simulink model "sldemo_wheelspeed_absbrake"  (R2020b)
settings: Solver=ode45  StartTime=0.0  StopTime=25  MaxStep=.01  RelTol=1e-3  AbsTol=1e-6
model workspace (MAT data in the model file):
  I = 5
  Kf = 1
  PBmax = 1500
  Rr = 1.25
  TB = 0.01
  v0 = 88
settings Model: ExtModeTrigMode=oneshot  ExtModeArmWhenConnect=off  ExtModeAutoUpdateStatusClock=off  Creator=WELCOME  LastModifiedBy=WELCOME
settings SolverCC: AutoScaleAbsTol=off
settings DataIOCC: SaveFormat=Array  SaveOutput=off  SaveTime=off  ReturnWorkspaceOutputs=off  TimeSaveName=time
settings OptimizationCC: DefaultParameterBehavior=Inlined  InlineInvariantSignals=on  ExpressionDepthLimit=2147483647  InitFltsAndDblsToZero=on  LifeSpan=inf  BufferReusableBoundary=off
settings DebuggingCC: SaveWithParameterizedLinksMsg=none  MultiTaskDSMMsg=warning  SigSpecEnsureSampleTimeMsg=none  IntegerOverflowMsg=none  FcnCallInpInsideContextMsg=warning  BusObjectLabelMismatch=none  ModelReferenceSymbolNameMessage=none  StateNameClashWarn=warning  SFUnexpectedBacktrackingDiag=warning  SFNoUnconditionalDefaultTransitionDiag=warning  SFExecutionAtInitializationDiag=none  IntegerSaturationMsg=none  ArithmeticOperatorsInVariantConditions=warning
settings HardwareCC: ProdBitPerPointer=32  ProdBitPerSizeT=32  ProdBitPerPtrDiffT=32  ProdLargestAtomicFloat=None  ProdIntDivRoundTo=Undefined  ProdEndianess=Unspecified  ProdWordSize=32  ProdHWDeviceType=32-bit Generic  TargetBitPerPointer=64  TargetBitPerSizeT=64  TargetBitPerPtrDiffT=64  TargetLongLongMode=on  TargetIntDivRoundTo=Zero  TargetEndianess=LittleEndian  TargetWordSize=64  TargetHWDeviceType=MATLAB Host
settings ModelReferenceCC: ModelReferenceMinAlgLoopOccurrences=on  PropagateSignalLabelsOutOfModel=off
settings SFSimCC: SimUseLocalCustomCode=off  CustomCodeUndefinedFunction=UseInterfaceOnly
settings RTWCC: Description=Rapid Simulation Target  SystemTargetFile=rsim.tlc  TemplateMakefile=rsim_default_tmf  RTWUseLocalCustomCode=off
settings CodeAppCC: StateflowObjectComments=on
settings RSimTargetCC: TargetFcnLib=ansi_tfl_tmw.mat
settings ConfigComp: CovMetricSettings=dw  CovSaveCumulativeToWorkspaceVar=on  CovSaveSingleToWorkspaceVar=on  CovExternalEMLEnable=off

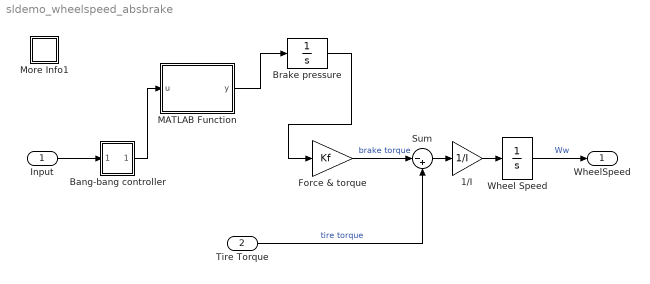
== system sldemo_wheelspeed_absbrake ==
  Input : Inport  SampleTime=0
  Tire Torque : Inport  Port=2
  1/I : Gain  Gain=1/I  SaturateOnIntegerOverflow=on  OutDataTypeStr=Inherit: Same as input  ParamDataTypeStr=Inherit: Same as input
  Bang-bang controller : Subsystem  mask(Sign){}
      mask help: y = sign(x)
      mask Help: Sign Function:\n\t\t\ty = 1 if x > 0\n\t\t\ty = 0 if x = 0\n\t\t\ty = -1 if x < 0
      mask Display: plot(-50,-50,50,50,[-50,50],[0,0],[0,0],[-50,50],[-40,0],[-30,-30],[0,40],[30,30])
  Brake pressure : Integrator  LimitOutput=on  UpperSaturationLimit=PBmax  LowerSaturationLimit=0
  Force & torque : Gain  Gain=Kf  SaturateOnIntegerOverflow=on  OutDataTypeStr=Inherit: Same as input  ParamDataTypeStr=Inherit: Same as input
  MATLAB Function : MATLAB Function  TreatAsAtomicUnit=on
  More Info1 : Subsystem
      settings: OpenFcn=showExample('simulink_automotive/ModelingAnAntiLockBrakingSystemExample')
      mask Display: disp('?')
  Sum : Sum  Inputs=|-+  InputSameDT=on  SaturateOnIntegerOverflow=on  OutDataTypeStr=Inherit: Same as first input
  Wheel Speed : Integrator  InitialCondition=v0/Rr  LimitOutput=on  UpperSaturationLimit=1000  LowerSaturationLimit=0
  WheelSpeed : Outport  VectorParamsAs1DForOutWhenUnconnected=off
  wires:
  1/I/1 -> Wheel Speed/1
  Sum/1 -> 1/I/1
  Force & torque/1 -> Sum/1  "brake torque"
  Brake pressure/1 -> Force & torque/1
  Bang-bang controller/1(out_1) -> MATLAB Function/1(u)
  MATLAB Function/1(y) -> Brake pressure/1
  Input/1 -> Bang-bang controller/1(in_1)
  Wheel Speed/1 -> WheelSpeed/1  "Ww"
  Tire Torque/1 -> Sum/2  "tire torque"

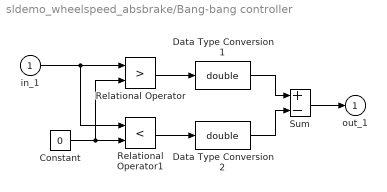
== system sldemo_wheelspeed_absbrake/Bang-bang controller ==
  in_1 : Inport
  Constant : Constant  Value=0
  Data Type Conversion1 : DataTypeConversion  OutDataTypeStr=double  SaturateOnIntegerOverflow=on  RndMeth=Zero
  Data Type Conversion2 : DataTypeConversion  OutDataTypeStr=double  SaturateOnIntegerOverflow=on  RndMeth=Zero
  Relational Operator : RelationalOperator  Operator=>  OutDataTypeStr=boolean  RndMeth=Nearest  InputSameDT=on
  Relational Operator1 : RelationalOperator  Operator=<  OutDataTypeStr=boolean  RndMeth=Nearest  InputSameDT=on
  Sum : Sum  Inputs=+-  InputSameDT=on  SaturateOnIntegerOverflow=on  OutDataTypeStr=Inherit: Same as first input
  out_1 : Outport  InitialOutput=0  VectorParamsAs1DForOutWhenUnconnected=off
  wires:
  Data Type Conversion2/1 -> Sum/2
  Data Type Conversion1/1 -> Sum/1
  Sum/1 -> out_1/1
  Relational Operator/1 -> Data Type Conversion1/1
  Relational Operator1/1 -> Data Type Conversion2/1
  Constant/1 -> Relational Operator/2, Relational Operator1/2
  in_1/1 -> Relational Operator1/1, Relational Operator/1

== system sldemo_wheelspeed_absbrake/More Info1 ==

== matlab function sldemo_wheelspeed_absbrake/MATLAB Function ==
  data: u input; y output
function y = fcn(u)

y = 100*u/(0.0100+1);
